simulink model "parameters_var"  (R2022a)
settings: Solver=ode3  StartTime=0.0  StopTime=2.5  FixedStep=1e-4  MaxStep=0.001  RelTol=1e-3
undefined symbols (not defined in the file): J, K1, K2, K3, K4, Ki, Ku, Lm, Lr, zp
libraries: simulink x1
settings Model: Creator=ver0sunny  LastModifiedBy=ver0sunny

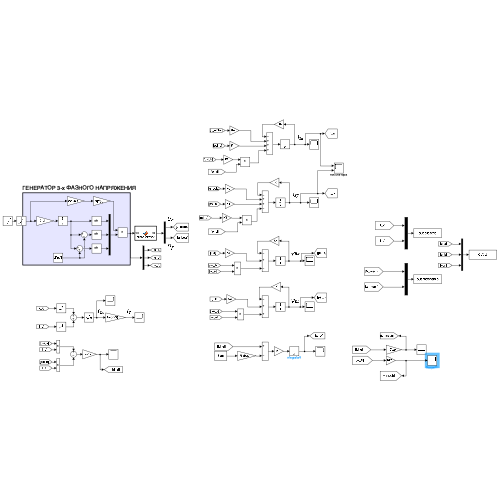
[thumbnail: Simulink's stored preview of the top-level diagram]
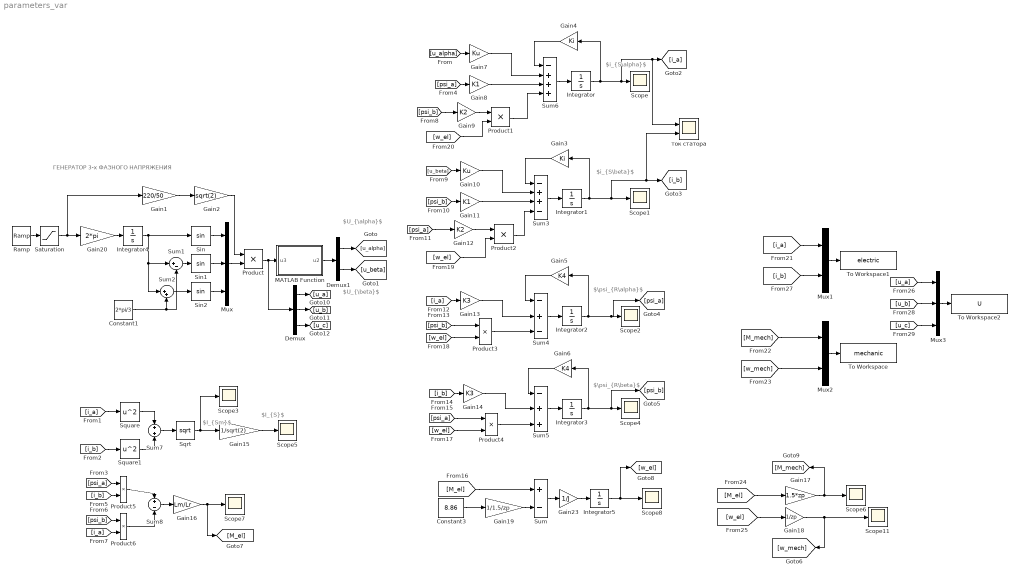
== system parameters_var ==
  note: $U_{\alpha}$
  note: ГЕНЕРАТОР 3-х ФАЗНОГО НАПРЯЖЕНИЯ
  note: $U_{\beta}$
  note: $i_{S\alpha}$
  note: $i_{S\beta}$
  note: $\psi_{R\alpha}$
  note: $\psi_{R\beta}$
  note: $I_{S}$
  note: $I_{Sm}$
  Constant1 : Constant  Value=2*pi/3
  Constant3 : Constant  Value=8.86
  Demux : Demux  Outputs=3
  Demux1 : Demux  Outputs=2
  Gain1 : Gain  Gain=220/50
  Gain10 : Gain  Gain=Ku
  Gain11 : Gain  Gain=K1
  Gain12 : Gain  Gain=K2
  Gain13 : Gain  Gain=K3
  Gain14 : Gain  Gain=K3
  Gain15 : Gain  Gain=1/sqrt(2)
  Gain16 : Gain  Gain=Lm/Lr
  Gain17 : Gain  Gain=1.5*zp
  Gain18 : Gain  Gain=1/zp
  Gain19 : Gain  Gain=1/1.5/zp
  Gain2 : Gain  Gain=sqrt(2)
  Gain20 : Gain  Gain=2*pi
  Gain23 : Gain  Gain=1/J
  Gain3 : Gain  Gain=Ki
  Gain4 : Gain  Gain=Ki
  Gain5 : Gain  Gain=K4
  Gain6 : Gain  Gain=K4
  Gain7 : Gain  Gain=Ku
  Gain8 : Gain  Gain=K1
  Gain9 : Gain  Gain=K2
  Integrator{,1..5} (6 alike) : Integrator
  MATLAB Function : MATLAB Function  TreatAsAtomicUnit=on
  Mux : Mux  Inputs=3
  Mux1 : Mux  Inputs=2
  Mux2 : Mux  Inputs=2
  Mux3 : Mux  Inputs=3
  Product{,1..6} (7 alike) : Product
  Ramp : simulink/Sources/Ramp  slope=150  start=0  InitialOutput=0.05*50
  Saturation : Saturate  UpperLimit=50  LowerLimit=0.05*50
  Scope{,1..8,11} (10 alike) : Scope
  Sin : Trigonometry
  Sin1 : Trigonometry
  Sin2 : Trigonometry
  Sqrt : Sqrt
  Square : Math  Operator=square
  Square1 : Math  Operator=square
  Sum : Sum  Inputs=+-
  Sum1 : Sum  Inputs=|+-
  Sum2 : Sum  Inputs=|++
  Sum3 : Sum  Inputs=-++-
  Sum4 : Sum  Inputs=-+-
  Sum5 : Sum  Inputs=-++
  Sum6 : Sum  Inputs=-+++
  Sum7 : Sum  Inputs=+|+
  Sum8 : Sum  Inputs=+|-
  To Workspace : ToWorkspace  VariableName=mechanic  SaveFormat=Timeseries  SampleTime=-1
  To Workspace1 : ToWorkspace  VariableName=electric  SaveFormat=Timeseries  SampleTime=-1
  To Workspace2 : ToWorkspace  VariableName=U  SaveFormat=Timeseries  SampleTime=-1
  ток статора : Scope  NumInputPorts=2
  wires:
  Integrator/1 -> ток статора/1, [i_a], Scope/1, Gain4/1
  Sin2/1 -> Mux/3
  Sin1/1 -> Mux/2
  Integrator4/1 -> Sum1/1, Sum2/1, Sin/1
  Sin/1 -> Mux/1
  Gain2/1 -> Product/1
  Mux/1 -> Product/2
  Sum2/1 -> Sin2/1
  Sum1/1 -> Sin1/1
  Constant1/1 -> Sum1/2, Sum2/2
  Gain1/1 -> Gain2/1
  Product/1 -> Demux/1, MATLAB Function/1(u3)
  MATLAB Function/1(u2) -> Demux1/1
  Demux1/1 -> [u_alpha]
  Demux1/2 -> [u_beta]
  Sum3/1 -> Integrator1/1
  Sum4/1 -> Integrator2/1
  Sum5/1 -> Integrator3/1
  Sum6/1 -> Integrator/1
  Gain4/1 -> Sum6/1
  Gain3/1 -> Sum3/1
  Integrator2/1 -> Gain5/1, [psi_a], Scope2/1
  Gain5/1 -> Sum4/1
  Integrator3/1 -> Gain6/1, [psi_b], Scope4/1
  Gain6/1 -> Sum5/1
  [u_alpha] -> Gain7/1
  Gain7/1 -> Sum6/2
  [psi_a] -> Gain8/1
  Gain8/1 -> Sum6/3
  [psi_b] -> Gain9/1
  [psi_a] -> Gain12/1
  Gain11/1 -> Sum3/3
  [psi_b] -> Gain11/1
  Gain10/1 -> Sum3/2
  [u_beta] -> Gain10/1
  [i_a] -> Gain13/1
  Gain13/1 -> Sum4/2
  [psi_b] -> Product3/1
  [psi_a] -> Product4/1
  Gain14/1 -> Sum5/2
  [i_b] -> Gain14/1
  Square1/1 -> Sum7/2
  Sum7/1 -> Sqrt/1
  Square/1 -> Sum7/1
  Gain15/1 -> Scope5/1
  Sqrt/1 -> Scope3/1, Gain15/1
  [i_a] -> Square/1
  [i_b] -> Square1/1
  [i_b] -> Product5/2
  [psi_a] -> Product5/1
  Product5/1 -> Sum8/1
  [psi_b] -> Product6/1
  [i_a] -> Product6/2
  Product6/1 -> Sum8/2
  Sum8/1 -> Gain16/1
  Product3/1 -> Sum4/3
  [M_el] -> Sum/1
  Sum/1 -> Gain23/1
  Gain23/1 -> Integrator5/1
  Integrator5/1 -> [w_el], Scope8/1
  Gain9/1 -> Product1/1
  Product1/1 -> Sum6/4
  Gain12/1 -> Product2/1
  Product2/1 -> Sum3/4
  Product4/1 -> Sum5/3
  [w_el] -> Product1/2
  [w_el] -> Product2/2
  [w_el] -> Product3/2
  [w_el] -> Product4/2
  Gain16/1 -> [M_el], Scope7/1
  Integrator1/1 -> Gain3/1, ток статора/2, [i_b], Scope1/1
  [M_mech] -> Mux2/1
  [w_mech] -> Mux2/2
  Mux2/1 -> To Workspace/1
  [w_el] -> Gain18/1
  Gain17/1 -> Scope6/1, [M_mech]
  [M_el] -> Gain17/1
  Gain18/1 -> Scope11/1, [w_mech]
  Constant3/1 -> Gain19/1
  Mux1/1 -> To Workspace1/1
  [i_a] -> Mux1/1
  [i_b] -> Mux1/2
  Demux/1 -> [u_a]
  Demux/2 -> [u_b]
  Demux/3 -> [u_c]
  [u_a] -> Mux3/1
  Mux3/1 -> To Workspace2/1
  [u_b] -> Mux3/2
  [u_c] -> Mux3/3
  Ramp/1 -> Saturation/1
  Saturation/1 -> Gain1/1, Gain20/1
  Gain20/1 -> Integrator4/1
  Gain19/1 -> Sum/2

== matlab function parameters_var/MATLAB Function ==
  data: u3 input; u2 output
function u2 = preobrazovat(u3)
    u2 = [2/3 -(1/3) -(1/3); 0 1/sqrt(3) -1/sqrt(3)] * u3;
end
